simulink model "New_vapourcontent"  (R2013b)
settings: Solver=FixedStepDiscrete  StartTime=0.0  StopTime=10  FixedStep=1  RelTol=1e-3
libraries: carnot x1
settings Model: Creator=awohlfei  LastModifiedBy=awohlfei
settings OptimizationCC: ExpressionDepthLimit=2147483647
settings DebuggingCC: UnderspecifiedInitializationDetection=Simplified  MergeDetectMultiDrivingBlocksExec=error  StateNameClashWarn=warning

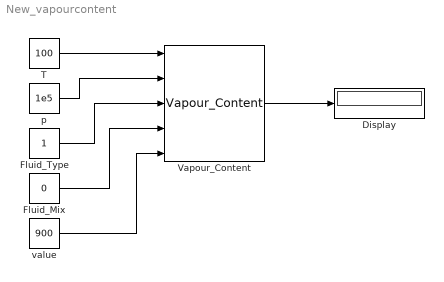
== system New_vapourcontent ==
  Display : Display
  Fluid_Mix : Constant  Value=0
  Fluid_Type : Constant
  T : Constant  Value=100
  Vapour_Content : carnot/Basic/Material_Properties/Vapour_Content  VariantControl=CarlibClassic  INPUTARGUMENTS=state variables (classic)  PROPERTYTYPE=density  DEBUGLEVEL=WARNINGLEVEL  MAXTOTALMESSAGES=inf  MAXCONSECUTIVEMESSAGES=inf  WRITETOFILE=0  FILENAME='errors.txt'
  p : Constant  Value=1e5
  value : Constant  Value=900
  wires:
  Vapour_Content/1 -> Display/1
  T/1 -> Vapour_Content/1
  p/1 -> Vapour_Content/2
  Fluid_Type/1 -> Vapour_Content/3
  Fluid_Mix/1 -> Vapour_Content/4
  value/1 -> Vapour_Content/5
